simulink model "SeparatelyExcited_model"  (R2024a)
settings: Solver=VariableStepAuto  StartTime=0.0  StopTime=50  RelTol=1e-3
undefined symbols (not defined in the file or in its folder): Bm3, dt, dT, Jm3, La3, Lf3, LoadMode, Ra3, Rf3, Ro, SlopeR, Ts, Vf3, Vp, Vs
libraries: simulink x1
settings Model: Creator=Xuan  LastModifiedBy=admin
settings RTWCC: GPUComputeCapability=3.5

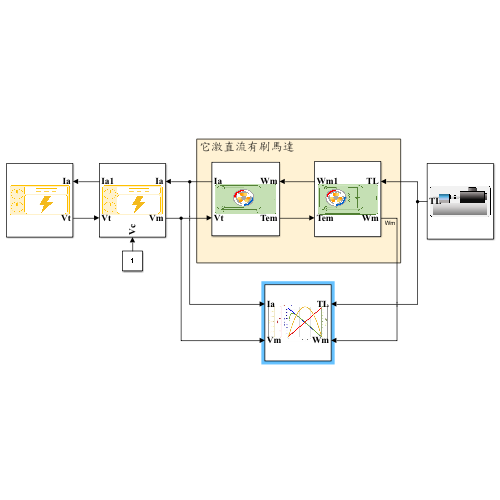
[thumbnail: Simulink's stored preview of the top-level diagram]
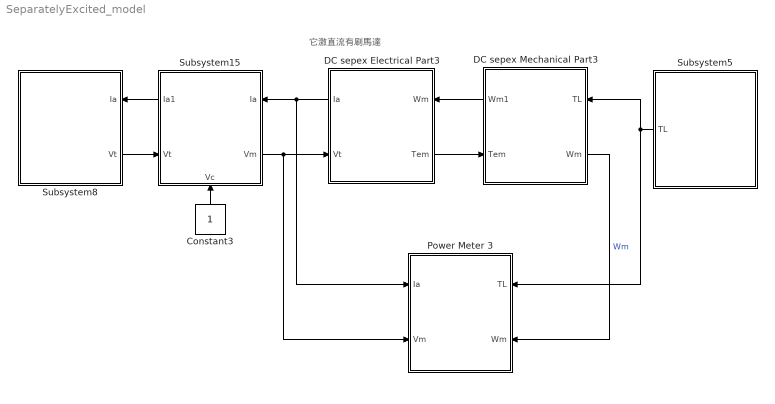
== system SeparatelyExcited_model ==
  note: 它激直流有刷馬達
  Constant3 : Constant
  DC sepex Electrical Part3 : Subsystem  InitFcn=|
      | La3 = 0.012;
      | Ra3 = 0.6;
      | Rf3 = 240;
      | Lf3 = 120;
      | Vf3 = 2;
      settings: PortSchema="{\"entries\":[{\"content\":{\"sides\":[{\"content\":{\"connectorIds\":[\"Out2\",\"In1\"]},\"type\":\"ConnectorPlacement.EquallySpacedRectSide\",\"uuid\":\"bcf8caf3-6f69-4504-a7ac-54864b04e584\"},{\"content\":{\"connectorIds\":[\"In2\",\"Out1\"],\"side\":\"RIGHT\"},\"type\":\"ConnectorPlacement.EquallySpacedRectSide\",\"uuid\":\"38d41819-7672-4c02-9170-774a5dddf0a6\"},{\"content\":{\"side\":\"TOP\"},\"type\":\"ConnectorPlacement.EquallySpacedRectSide\",\"uuid\":\"ec4d207e-12b8-4ef5-9f8a-a31af86c34d6\"},{\"content\":{\"side\":\"BOTTOM\"},\"type\":\"ConnectorPlacement.EquallySpacedRectSide\",\"uuid\":\"e747e378-c395-4326-997f-7ad970ad93b7\"}]},\"type\":\"ConnectorPlacement.EquallySpacedConnector\",\"uuid\":\"43deb926-5ff2-4c5e-a4ab-89e47786c42d\"}],\"packageUris\":[\"http://schema.mathworks.com/mf0/Connector/R2020b\"],\"version\":\"1.0\"}"
      mask Display: image('直流它激馬達2.png');
  DC sepex Mechanical Part3 : Subsystem  InitFcn=|
      | Jm3 = 1;
      | Bm3 = 0.02;
      settings: PortSchema="{\"entries\":[{\"content\":{\"sides\":[{\"content\":{\"connectorIds\":[\"Out2\",\"In1\"]},\"type\":\"ConnectorPlacement.EquallySpacedRectSide\",\"uuid\":\"aa24ada9-515e-4cdb-a8da-2d886abb389d\"},{\"content\":{\"connectorIds\":[\"In2\",\"Out1\"],\"side\":\"RIGHT\"},\"type\":\"ConnectorPlacement.EquallySpacedRectSide\",\"uuid\":\"72599521-268d-4a0b-847e-8595f852538d\"},{\"content\":{\"connectorIds\":[],\"side\":\"TOP\"},\"type\":\"ConnectorPlacement.EquallySpacedRectSide\",\"uuid\":\"7aa775e0-56de-4d39-8fe3-ba0ef8ecc165\"}]},\"type\":\"ConnectorPlacement.EquallySpacedConnector\",\"uuid\":\"0b47bd83-24f5-4cc4-a2dd-91de7f957050\"}],\"packageUris\":[\"http://schema.mathworks.com/mf0/Connector/R2020b\"],\"version\":\"1.0\"}"
      mask Display: image('直流它激馬達2.png');
  Power Meter 3 : Subsystem  InitFcn=|  StopFcn=|
      InitFcn=|
      | %% ModePlot
      | % PlotMode=1 or 2
      | PlotMode = 2;
      StopFcn=|
      | % %% Data Loading
      | % 
      | % tl3 = out.Tl3;
      | % f3 = size(tl3);
      | % 
      | % % clear datas 
      | % torque3 = 0;
      | % x13 = 0;
      | % y13 = 0; y23 = 0; y33 = 0; y43 = 0; y53 = 0; y63 = 0;
      | % 
      | % switch LoadMode   % mode ( 1:ramp load , 2:stair load )
      | % 
      | %     case 1  
      | % 
      | %         i = 1;
      | %         while 1
      | %             if tl3(i) > 0.01
      | %                s = i;
      | %                break
      | %             end
      | %             i = i+1;
      | %         end
      | %         torque3 = out.Tl3(s:f3(1));
      | %         x13 = out.omega3(s:f3(1));
      | %         % y13 = out.omega3(s:f3(1));
      | %         y23 = out.Eff3(s:f3(1));
      | %         y33 = out.Pin3(s:f3(1));
      | %         y43 = out.Pout3(s:f3(1));
      | %         y53 = out.Vs(s:f3(1));
      | %         y63 = out.Ia3(s:f3(1));
      | %         case 2
      | % 
      | %         tl_pre3 = 0;
      | %         j = 1;
      | %         for i = 1:f3(1)           
      | %             if tl3(i) > tl_pre3
      | %                 torque3(j,1) = tl3(i-1);
      | %                 x13(j,1) = out.omega3((i-1),1);
      | %                 % y13(j,1) = out.omega3((i-1),1);
      | %                 y23(j,1) = out.Eff3((i-1),1);
      | %                 y33(j,1) = out.Pin3((i-1),1);
      | %                 y43(j,1) = out.Pout3((i-1),1);
      | %                 y53(j,1) = out.Vs((i-1),1);
      | %                 y63(j,1) = out.Ia3((i-1),1);
      | %                 j = j+1;
      | %             end
      | %             tl_pre3 = tl3(i);
      | %         end
      | % end
      | % 
      | % %% Plot
      | % % plot TN curve
      | % 
      | % % figure(1);
      | % 
      | % figure(4);
      | % set(gcf, 'Position', [1050, 300, 1000, 500]); % [left, bottom, width, height]
      | % clf;
      | % 
      | % % Create empty axis system with 4 y axis by calling:
      | % % handle = maxis(number of axis, y-spacing between outside lines)
      | % h = myaxisc(5,0.10,[0.1,0.1,0.8,0.8]); % Specify position
      | % 
      | % % Call plot and specify y-axis number using method h.p(nr). For creating a
      | % % legend later, we need to assign the handles returned by plot to p.
      | % switch PlotMode
      | % 
      | %     case 1  
      | %         p(1) = plot(h.p(1),x13,torque3,'b','LineWidth',1.2);
      | %         p(2) = plot(h.p(2),x13,y23,'Color',[0.4660 0.6740 0.1880],'LineWidth',1.2);
      | %         p(3) = plot(h.p(3),x13,y63,'Color',[0.3010 0.7450 0.9330],'LineWidth',1.2);
      | %         p(4) = plot(h.p(4),x13,y53,'r','LineWidth',1.2);
      | %         p(5) = plot(h.p(5),x13,y33,'m','LineWidth',1.2);
      | %         print("case1");
      | % 
      | %     case 2
      | %         p(1) = plot(h.p(1),x13,torque3,'b-*','LineWidth',1.1);
      | %         p(2) = plot(h.p(2),x13,y23,'-*','Color',[0.4660 0.6740 0.1880],'LineWidth',1.1);
      | %         p(3) = plot(h.p(3),x13,y63,'-*','Color',[0.3010 0.7450 0.9330],'LineWidth',1.1);
      | %         p(4) = plot(h.p(4),x13,y53,'r-*','LineWidth',1.1);
      | %         p(5) = plot(h.p(5),x13,y33,'m-*','LineWidth',1.1);
      | %         print("case2");
      | % 
      | % end
      | % 
      | % h.autoscale % Automatically Scale Y Axis
      | % 
      | % % Additional methods to modify appearance, scaling and so on:
      | % 
      | % h.autoy(3) % Autoscale only specified y-axis
      | % %h.ylim(3,[95,105]); % Set Y-Limits for axis 3
      | % l3 = size(torque3);
      | % h.xlim([min(x13),max(x13)]);
      | % h.ylim(2,[0,100]); % Set Y-Limits for axis 4
      | % 
      | % h.gridon % Enable grid (use h.gridoff to remove)
      | % 
      | % % Modify the y-Axis Color
      | % h.ycolor(1,'b'); % torque
      | % h.ycolor(2,[0.4660 0.6740 0.1880]); % efficiency
      | % h.ycolor(3,[0.3010 0.7450 0.9330]); % current
      | % h.ycolor(4,'r'); % voltage
      | % h.ycolor(5,'m'); % power in
      | % 
      | % % Add y-Labels
      | % % h.ylabel(1,'Speed (RPM)');
      | % h.ylabel(1, 'TL (Nm)');
      | % h.ylabel(2,'Efficiency (%)');
      | % h.ylabel(3,'Current (A)');
      | % h.ylabel(4,'Voltage (volt)');
      | % h.ylabel(5,'Pin (W)');
      | % 
      | % % Add x-Label
      | % % h.xlabel('TL (Nm)');
      | % h.xlabel('Speed (RPM)');
      | % 
      | % % Add title
      | % title('TNcurve of Separately Excited Motor');
      | % set(gca,'FontWeight','bold','FontSize',14);
      | % 
      | % % Change Position of the whole myaxisc-Object
      | % h.position([0.1,0.1,0.8,0.8],0.12); % Position-Vector and Spacing 0.12
      | % 
      | % % Change all font sizes
      | % h.fontsize(10)
      | % 
      | % %% DataSaving
      | % time = out.tout;
      | % powerin3 = out.Pin3;
      | % powerout3 = out.Pout3;
      | % speed3 = out.omega3;
      | % efficiency3 = out.Eff3;
      | % voltage3 = out.Vs;
      | % current3 = out.Ia3;
      | % 
      | % filename = 'Seperately_TNcurve_DataSave.csv';
      | % savedata = [time, powerin3, powerout3, speed3, efficiency3, voltage3, current3];
      | % writematrix(savedata, filename);
      settings: PortSchema="{\"entries\":[{\"content\":{\"sides\":[{\"content\":{\"connectorIds\":[\"In1\",\"In2\"]},\"type\":\"ConnectorPlacement.EquallySpacedRectSide\",\"uuid\":\"e8c36156-32d4-4676-af0d-0891e0773ccb\"},{\"content\":{\"connectorIds\":[\"In3\",\"In4\"],\"side\":\"RIGHT\"},\"type\":\"ConnectorPlacement.EquallySpacedRectSide\",\"uuid\":\"5c876be3-b715-4990-b5f5-1fbda74411c9\"},{\"content\":{\"side\":\"TOP\"},\"type\":\"ConnectorPlacement.EquallySpacedRectSide\",\"uuid\":\"8aaa78a6-3767-49bf-860f-056d8a2101ef\"}]},\"type\":\"ConnectorPlacement.EquallySpacedConnector\",\"uuid\":\"6a38af7a-9eb4-49af-a88b-27cf70b05ead\"}],\"packageUris\":[\"http://schema.mathworks.com/mf0/Connector/R2020b\"],\"version\":\"1.0\"}"
      mask Display: image('TNcurve2.png');
  Subsystem15 : Subsystem  InitFcn=Vp = 1;
      settings: PortSchema="{\"entries\":[{\"content\":{\"sides\":[{\"content\":{\"connectorIds\":[\"Out2\",\"In1\"]},\"type\":\"ConnectorPlacement.EquallySpacedRectSide\",\"uuid\":\"717e91a0-288b-4ba5-84da-f262c24688bc\"},{\"content\":{\"connectorIds\":[\"In3\",\"Out1\"],\"side\":\"RIGHT\"},\"type\":\"ConnectorPlacement.EquallySpacedRectSide\",\"uuid\":\"569ee505-38fb-400b-9e45-0fafedafb0f3\"},{\"content\":{\"side\":\"TOP\"},\"type\":\"ConnectorPlacement.EquallySpacedRectSide\",\"uuid\":\"44407c3d-239d-4fc9-b2d2-10ddbad2f525\"},{\"content\":{\"connectorIds\":[\"In2\"],\"side\":\"BOTTOM\"},\"type\":\"ConnectorPlacement.EquallySpacedRectSide\",\"uuid\":\"abc944a0-1837-407a-a5f0-1c34ab870232\"}]},\"type\":\"ConnectorPlacement.EquallySpacedConnector\",\"uuid\":\"e894aa65-7991-48d5-91da-50bab94327d3\"}],\"packageUris\":[\"http://schema.mathworks.com/mf0/Connector/R2020b\"],\"version\":\"1.0\"}"
      mask Display: image('直流電源2.png');
  Subsystem5 : Subsystem  InitFcn=|
      | dt = 0.2;
      | dT = 0.05;
      | Ts = 2;
      | SlopeR = 0.2;
      | % if LoadMode>1.5, then use stair load
      | % if LoadMode<1.5, use linear load
      | LoadMode = 2;
      mask Display: image('主動式動力機2.png');
  Subsystem8 : Subsystem  InitFcn=|
      | Vs = 220;
      | Ro = 0.001;
      settings: PortSchema="{\"entries\":[{\"content\":{\"sides\":[{\"content\":{},\"type\":\"ConnectorPlacement.EquallySpacedRectSide\",\"uuid\":\"717e91a0-288b-4ba5-84da-f262c24688bc\"},{\"content\":{\"connectorIds\":[\"In1\",\"Out1\"],\"side\":\"RIGHT\"},\"type\":\"ConnectorPlacement.EquallySpacedRectSide\",\"uuid\":\"569ee505-38fb-400b-9e45-0fafedafb0f3\"},{\"content\":{\"side\":\"TOP\"},\"type\":\"ConnectorPlacement.EquallySpacedRectSide\",\"uuid\":\"44407c3d-239d-4fc9-b2d2-10ddbad2f525\"}]},\"type\":\"ConnectorPlacement.EquallySpacedConnector\",\"uuid\":\"e894aa65-7991-48d5-91da-50bab94327d3\"}],\"packageUris\":[\"http://schema.mathworks.com/mf0/Connector/R2020b\"],\"version\":\"1.0\"}"
      mask Display: image('直流電源2.png', "center");
  wires:
  DC sepex Mechanical Part3/1(Wm) -> Power Meter 3/4(Wm)  "Wm"
  DC sepex Electrical Part3/2(Ia) -> Subsystem15/3(Ia), Power Meter 3/1(Ia)
  DC sepex Electrical Part3/1(Tem) -> DC sepex Mechanical Part3/1(Tem)
  DC sepex Mechanical Part3/2(Wm1) -> DC sepex Electrical Part3/2(Wm)
  Subsystem15/2(Ia1) -> Subsystem8/1(Ia)
  Subsystem8/1(Vt) -> Subsystem15/1(Vt)
  Subsystem15/1(Vm) -> Power Meter 3/2(Vm), DC sepex Electrical Part3/1(Vt)
  Subsystem5/1(TL) -> DC sepex Mechanical Part3/2(TL), Power Meter 3/3(TL)
  Constant3/1 -> Subsystem15/2(Vc)

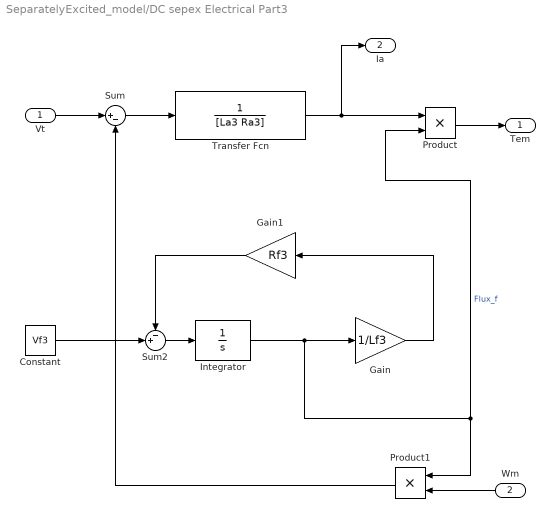
== system SeparatelyExcited_model/DC sepex Electrical Part3 ==
  Vt : Inport
  Wm : Inport  Port=2
  Constant : Constant  Value=Vf3
  Gain : Gain  Gain=1/Lf3
  Gain1 : Gain  Gain=Rf3
  Integrator : Integrator
  Product : Product
  Product1 : Product
  Sum : Sum  Inputs=|+-
  Sum2 : Sum  Inputs=-+|
  Transfer Fcn : TransferFcn  Denominator=[La3 Ra3]
  Tem : Outport
  Ia : Outport  Port=2
  wires:
  Wm/1 -> Product1/2
  Vt/1 -> Sum/1
  Product/1 -> Tem/1
  Constant/1 -> Sum2/2
  Transfer Fcn/1 -> Product/1, Ia/1
  Sum/1 -> Transfer Fcn/1
  Sum2/1 -> Integrator/1
  Integrator/1 -> Gain/1, Product1/1, Product/2  "Flux_f"
  Gain/1 -> Gain1/1
  Gain1/1 -> Sum2/1
  Product1/1 -> Sum/2

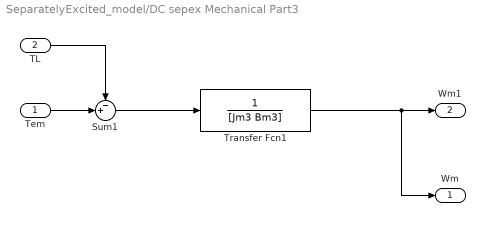
== system SeparatelyExcited_model/DC sepex Mechanical Part3 ==
  Tem : Inport
  TL : Inport  Port=2
  Sum1 : Sum  Inputs=-+|
  Transfer Fcn1 : TransferFcn  Denominator=[Jm3 Bm3]
  Wm : Outport
  Wm1 : Outport  Port=2
  wires:
  Tem/1 -> Sum1/2
  TL/1 -> Sum1/1
  Sum1/1 -> Transfer Fcn1/1
  Transfer Fcn1/1 -> Wm1/1, Wm/1

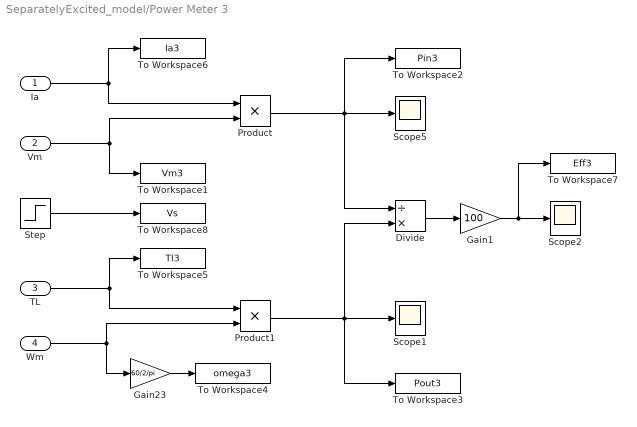
== system SeparatelyExcited_model/Power Meter 3 ==
  Ia : Inport
  Vm : Inport  Port=2
  TL : Inport  Port=3
  Wm : Inport  Port=4
  Divide : Product  Inputs=/*
  Gain1 : Gain  Gain=100
  Gain23 : Gain  Gain=60/2/pi
  Product : Product
  Product1 : Product
  Scope1 : Scope
  Scope2 : Scope
  Scope5 : Scope
  Step : Step  Time=0.1  After=Vs  SampleTime=0
  To Workspace1 : ToWorkspace  VariableName=Vm3  SampleTime=-1
  To Workspace2 : ToWorkspace  VariableName=Pin3  SampleTime=-1
  To Workspace3 : ToWorkspace  VariableName=Pout3  SampleTime=-1
  To Workspace4 : ToWorkspace  VariableName=omega3  SampleTime=-1
  To Workspace5 : ToWorkspace  VariableName=Tl3  SampleTime=-1
  To Workspace6 : ToWorkspace  VariableName=Ia3  SampleTime=-1
  To Workspace7 : ToWorkspace  VariableName=Eff3  SampleTime=-1
  To Workspace8 : ToWorkspace  VariableName=Vs  SampleTime=-1
  wires:
  Gain1/1 -> Scope2/1, To Workspace7/1
  Divide/1 -> Gain1/1
  Gain23/1 -> To Workspace4/1
  Wm/1 -> Gain23/1, Product1/2
  TL/1 -> Product1/1, To Workspace5/1
  Product1/1 -> Divide/2, To Workspace3/1, Scope1/1
  Product/1 -> To Workspace2/1, Scope5/1, Divide/1
  Vm/1 -> Product/2, To Workspace1/1
  Ia/1 -> To Workspace6/1, Product/1
  Step/1 -> To Workspace8/1

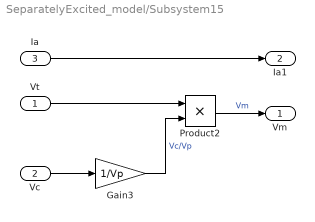
== system SeparatelyExcited_model/Subsystem15 ==
  Vt : Inport
  Vc : Inport  Port=2
  Ia : Inport  Port=3
  Gain3 : Gain  Gain=1/Vp
  Product2 : Product
  Vm : Outport
  Ia1 : Outport  Port=2
  wires:
  Gain3/1 -> Product2/2  "Vc/Vp"
  Product2/1 -> Vm/1  "Vm"
  Vt/1 -> Product2/1
  Vc/1 -> Gain3/1
  Ia/1 -> Ia1/1

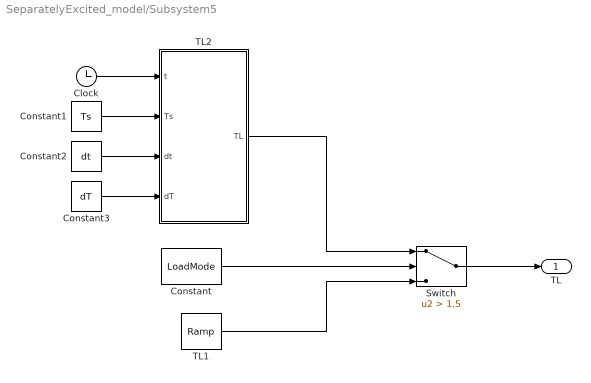
== system SeparatelyExcited_model/Subsystem5 ==
  Clock : Clock
  Constant : Constant  Value=LoadMode
  Constant1 : Constant  Value=Ts
  Constant2 : Constant  Value=dt  SampleTime=dT
  Constant3 : Constant  Value=dT
  Switch : Switch  Criteria=u2 > Threshold  Threshold=1.5  SaturateOnIntegerOverflow=off  InputSameDT=off
  TL1 : simulink/Sources/Ramp  slope=SlopeR  start=Ts  InitialOutput=0
  TL2 : MATLAB Function  TreatAsAtomicUnit=on
  TL : Outport
  wires:
  TL1/1 -> Switch/3
  TL2/1(TL) -> Switch/1
  Constant/1 -> Switch/2
  Switch/1 -> TL/1
  Constant1/1 -> TL2/2(Ts)
  Clock/1 -> TL2/1(t)
  Constant3/1 -> TL2/4(dT)
  Constant2/1 -> TL2/3(dt)

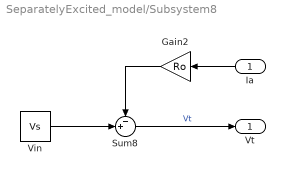
== system SeparatelyExcited_model/Subsystem8 ==
  Ia : Inport
  Gain2 : Gain  Gain=Ro
  Sum8 : Sum  Inputs=-+|
  Vin : Constant  Value=Vs
  Vt : Outport
  wires:
  Ia/1 -> Gain2/1
  Vin/1 -> Sum8/2
  Sum8/1 -> Vt/1  "Vt"
  Gain2/1 -> Sum8/1

== matlab function SeparatelyExcited_model/Subsystem5/TL2 ==
  data: t input; Ts input; TL output; dt input; dT input
function TL = fcn(t, Ts, dt, dT)

if t >= Ts
        TL = dT * fix((t-Ts)/dt);
else
    TL = 0;
end
